simulink subsystem "RW"  (R2025b)
settings: Solver=VariableStepAuto  StartTime=0.0  StopTime=10.0  RelTol=1e-3
model mask{rwInertia=0, rwMaxOmg=0, rwMaxTorque=0, rwInitOmg=0}
  mask prompts: rwInertia "Inertia moment [kgm-1]"; rwMaxOmg "Maximum angular velocity [rads-1]"; rwMaxTorque "Maximum torque [Nm]"; rwInitOmg "Initial angular velocity [rads-1]"
settings Model: Creator=antoniohernandez-rodiciomateos  LastModifiedBy=antoniohernandez-rodiciomateos

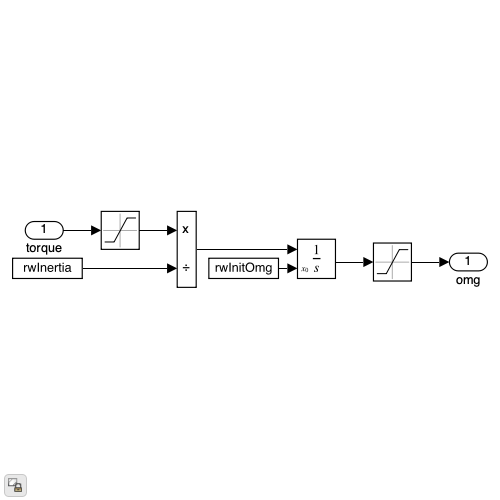
[thumbnail: Simulink's stored preview of the top-level diagram]
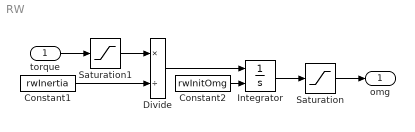
== system RW ==
  torque : Inport  OutDataTypeStr=double  PortDimensions=[1 1]
  Constant1 : Constant  Value=rwInertia
  Constant2 : Constant  Value=rwInitOmg
  Divide : Product  Inputs=*/
  Integrator : Integrator  InitialConditionSource=external
  Saturation : Saturate  UpperLimit=rwMaxOmg  LowerLimit=-1 * rwMaxOmg
  Saturation1 : Saturate  UpperLimit=rwMaxTorque  LowerLimit=-1 * rwMaxTorque
  omg : Outport
  wires:
  Constant1/1 -> Divide/2
  Divide/1 -> Integrator/1
  Constant2/1 -> Integrator/2
  Integrator/1 -> Saturation/1
  Saturation/1 -> omg/1
  Saturation1/1 -> Divide/1
  torque/1 -> Saturation1/1
